simulink model "eVTOL_System"  (R2024b)
settings: Solver=FixedStepAuto  StartTime=0.0  StopTime=inf  RelTol=1e-3
undefined symbols (not defined in the file): airspeed, Battery, BCE12, BCE_Set_init, BMS_Controller_State, C, Cell10_P, Cell11_P, Cell12_P, Cell13_P, Cell14_P, Cell15_P, Cell16_P, Cell17_P, Cell18_P, Cell19_P, Cell1_N, Cell1_P, Cell20_P, Cell21_P, Cell22_P, Cell23_P, Cell24_P, Cell2_P, Cell3_P, Cell4_P, Cell5_P, Cell6_P, Cell7_P, Cell8_P, Cell9_P, Charging_State, CityMission, control, controlParams, ControlSampleTime, CriticalTiltAngle, currentFactor, CV_Gain, ddx, ddy, ddz, Device_01, Device_02, DiscIntNeverNeededParam, dx, dy, dz, Earth, env, F, F28379D_ADC_MaxCount, F28379D_ADC_Vmax, FixedWingMission, flightState, Foc_Ki_IxTcpu, Foc_Ki_S, Foc_Kp_I, Foc_Kp_S, fractalcoef ... (+68)
libraries: fl_lib x1115, nesl_utility x617, slrealtimeethercatlib x217, simulink x130, canmsglib x101, speedgoatlib_IO611_obsolete x91, slpidlib x49, mcbcontrolslib x44, slrealtimeutilitieslib x35, speedgoatlib_hdlCoder_IO3xx x31, dspstat3 x24, mcbpositiondecoderlib x12
(part 14 of 31)

== system eVTOL_System/Motor Drive/Controller1/Controller_MIL/F28379D Firmware/Phase_Current_Rescaling ==
  Ia_ADC : Inport
  Ib_ADC : Inport  Port=2
  IaOffset : Inport  Port=3
  IbOffset : Inport  Port=4
  ADCtoA : Gain  Gain=10/IO334_DAC_Vmax/IO334_iDAC_gain  RndMeth=Simplest  OutDataTypeStr=Inherit: Same as input
  Add : Sum  Inputs=+-
  Add Constant : Bias  Bias=-2^11*IO334_DAC_Vmax/F28379D_ADC_Vmax  SaturateOnIntegerOverflow=off
  Get ADC Voltage : Gain  Gain=F28379D_ADC_Vmax/F28379D_ADC_MaxCount  OutDataTypeStr=single  RndMeth=Simplest
  Mux : Mux  Inputs=2
  Mux1 : Mux  Inputs=2
  PU_Conversion : Gain  Gain=1/PU_System_I_base  RndMeth=Simplest  OutDataTypeStr=Inherit: Same as input
  Rate Transition : RateTransition
  Iab_meas_PU : Outport  VectorParamsAs1DForOutWhenUnconnected=off
  wires:
  Mux1/1 -> Rate Transition/1
  Ia_ADC/1 -> Mux/1
  Ib_ADC/1 -> Mux/2
  Mux/1 -> Add Constant/1
  PU_Conversion/1 -> Iab_meas_PU/1
  IaOffset/1 -> Mux1/1
  IbOffset/1 -> Mux1/2
  Add Constant/1 -> Get ADC Voltage/1
  Get ADC Voltage/1 -> ADCtoA/1  "Currents_inDACvoltages"
  Rate Transition/1 -> Add/2
  ADCtoA/1 -> Add/1  "Currents_A"
  Add/1 -> PU_Conversion/1  "Currents_no_offset"

== system eVTOL_System/Motor Drive/Controller1/Controller_MIL/F28379D Firmware/Speed Conditioning ==
  Spd[rpm] : Inport
  hz2pu : Gain  Gain=60/(PU_System_N_base *Maxon_645604_Np)  RndMeth=Simplest  OutDataTypeStr=Inherit: Same as input
  rads2hz : Gain  Gain=Maxon_645604_Np/(2*pi)
  rmp2rads : Gain  Gain=2*pi/60
  Spd[PU] : Outport
  wires:
  Spd[rpm]/1 -> rmp2rads/1
  rmp2rads/1 -> rads2hz/1
  rads2hz/1 -> hz2pu/1
  hz2pu/1 -> Spd[PU]/1

== system eVTOL_System/Motor Drive/Controller2/Controller_MIL/F28379D Firmware/Controller Algorithm ==
  Ia_PU : Inport
  QEP_Position_Count : Inport  Port=2
  QEP_Index_Latch : Inport  Port=3
  SpdCmd : Inport  Port=4
  Kp_S : Inport  Port=5
  Ki_S : Inport  Port=6
  EnClosedLoop : Inport  Port=7
  EnablePWM : Inport  Port=8
  Kp_i : Inport  Port=9
  Ki_ixTcpu : Inport  Port=10
  AND : Logic  IconShape=distinctive  AllPortsSameDT=off  OutDataTypeStr=boolean
  Data Type Conversion : DataTypeConversion  OutDataTypeStr=single  SaturateOnIntegerOverflow=off  RndMeth=Floor
  Demux : Demux  Outputs=2
  FOC : Subsystem
  Gain : Gain  Gain=PU_System_I_base
  Gain1 : Gain  Gain=PU_System_N_base
  Mux : Mux  Inputs=2
  Speed and Pos Decoder : Subsystem
  pmsm.PositionOffset : Constant  Value=0  SampleTime=-1
  ModWave : Outport
  PWM_Enable : Outport  Port=2
  fbk_CAN : Outport  Port=3
  wires:
  EnClosedLoop/1 -> AND/2
  Speed and Pos Decoder/1(Theta_e) -> FOC/2(Pos)
  Ia_PU/1 -> FOC/1(Iab), Gain/1
  EnablePWM/1 -> FOC/6(EnablePWM)
  Speed and Pos Decoder/3(IndexFound) -> AND/1
  AND/1 -> FOC/4(EnClosedLoop)
  pmsm.PositionOffset/1 -> Speed and Pos Decoder/3(Offset)
  Speed and Pos Decoder/2(speed) -> FOC/3(Speedfb), Gain1/1
  FOC/2(PWM_Enable) -> PWM_Enable/1
  QEP_Index_Latch/1 -> Speed and Pos Decoder/2(QEP_Index_Latch)
  FOC/1(ModWave) -> ModWave/1  "ModWave"
  Kp_S/1 -> FOC/7(Kp_S)
  Ki_S/1 -> FOC/8(Ki_S)
  SpdCmd/1 -> FOC/5(SpeedRef)
  [Speed] -> Mux/1
  [Pos] -> Mux/2
  Mux/1 -> fbk_CAN/1
  Demux/1 -> [Ia_PU]
  Demux/2 -> [Ib_PU]
  Kp_i/1 -> FOC/9(Kp_i)
  Ki_ixTcpu/1 -> FOC/10(Ki_ixTcpu)
  Gain/1 -> Demux/1
  Gain1/1 -> [Speed]
  QEP_Position_Count/1 -> Speed and Pos Decoder/1(QEP_Position_Count), Data Type Conversion/1
  Data Type Conversion/1 -> [Pos]

== system eVTOL_System/Motor Drive/Controller2/Controller_MIL/F28379D Firmware/Phase_Current_Rescaling ==
  Ia_ADC : Inport
  Ib_ADC : Inport  Port=2
  IaOffset : Inport  Port=3
  IbOffset : Inport  Port=4
  ADCtoA : Gain  Gain=10/IO334_DAC_Vmax/IO334_iDAC_gain  RndMeth=Simplest  OutDataTypeStr=Inherit: Same as input
  Add : Sum  Inputs=+-
  Add Constant : Bias  Bias=-2^11*IO334_DAC_Vmax/F28379D_ADC_Vmax  SaturateOnIntegerOverflow=off
  Get ADC Voltage : Gain  Gain=F28379D_ADC_Vmax/F28379D_ADC_MaxCount  OutDataTypeStr=single  RndMeth=Simplest
  Mux : Mux  Inputs=2
  Mux1 : Mux  Inputs=2
  PU_Conversion : Gain  Gain=1/PU_System_I_base  RndMeth=Simplest  OutDataTypeStr=Inherit: Same as input
  Rate Transition : RateTransition
  Iab_meas_PU : Outport  VectorParamsAs1DForOutWhenUnconnected=off
  wires:
  Mux1/1 -> Rate Transition/1
  Ia_ADC/1 -> Mux/1
  Ib_ADC/1 -> Mux/2
  Mux/1 -> Add Constant/1
  PU_Conversion/1 -> Iab_meas_PU/1
  IaOffset/1 -> Mux1/1
  IbOffset/1 -> Mux1/2
  Add Constant/1 -> Get ADC Voltage/1
  Get ADC Voltage/1 -> ADCtoA/1  "Currents_inDACvoltages"
  Rate Transition/1 -> Add/2
  ADCtoA/1 -> Add/1  "Currents_A"
  Add/1 -> PU_Conversion/1  "Currents_no_offset"

== system eVTOL_System/Motor Drive/Controller2/Controller_MIL/F28379D Firmware/Speed Conditioning ==
  Spd[rpm] : Inport
  hz2pu : Gain  Gain=60/(PU_System_N_base *Maxon_645604_Np)  RndMeth=Simplest  OutDataTypeStr=Inherit: Same as input
  rads2hz : Gain  Gain=Maxon_645604_Np/(2*pi)
  rmp2rads : Gain  Gain=2*pi/60
  Spd[PU] : Outport
  wires:
  Spd[rpm]/1 -> rmp2rads/1
  rmp2rads/1 -> rads2hz/1
  rads2hz/1 -> hz2pu/1
  hz2pu/1 -> Spd[PU]/1

== system eVTOL_System/Motor Drive/Controller3/Controller_MIL/F28379D Firmware/Controller Algorithm ==
  Ia_PU : Inport
  QEP_Position_Count : Inport  Port=2
  QEP_Index_Latch : Inport  Port=3
  SpdCmd : Inport  Port=4
  Kp_S : Inport  Port=5
  Ki_S : Inport  Port=6
  EnClosedLoop : Inport  Port=7
  EnablePWM : Inport  Port=8
  Kp_i : Inport  Port=9
  Ki_ixTcpu : Inport  Port=10
  AND : Logic  IconShape=distinctive  AllPortsSameDT=off  OutDataTypeStr=boolean
  Data Type Conversion : DataTypeConversion  OutDataTypeStr=single  SaturateOnIntegerOverflow=off  RndMeth=Floor
  Demux : Demux  Outputs=2
  FOC : Subsystem
  Gain : Gain  Gain=PU_System_I_base
  Gain1 : Gain  Gain=PU_System_N_base
  Mux : Mux  Inputs=2
  Speed and Pos Decoder : Subsystem
  pmsm.PositionOffset : Constant  Value=0  SampleTime=-1
  ModWave : Outport
  PWM_Enable : Outport  Port=2
  fbk_CAN : Outport  Port=3
  wires:
  EnClosedLoop/1 -> AND/2
  Speed and Pos Decoder/1(Theta_e) -> FOC/2(Pos)
  Ia_PU/1 -> FOC/1(Iab), Gain/1
  EnablePWM/1 -> FOC/6(EnablePWM)
  Speed and Pos Decoder/3(IndexFound) -> AND/1
  AND/1 -> FOC/4(EnClosedLoop)
  pmsm.PositionOffset/1 -> Speed and Pos Decoder/3(Offset)
  Speed and Pos Decoder/2(speed) -> FOC/3(Speedfb), Gain1/1
  FOC/2(PWM_Enable) -> PWM_Enable/1
  QEP_Index_Latch/1 -> Speed and Pos Decoder/2(QEP_Index_Latch)
  FOC/1(ModWave) -> ModWave/1  "ModWave"
  Kp_S/1 -> FOC/7(Kp_S)
  Ki_S/1 -> FOC/8(Ki_S)
  SpdCmd/1 -> FOC/5(SpeedRef)
  [Speed] -> Mux/1
  [Pos] -> Mux/2
  Mux/1 -> fbk_CAN/1
  Demux/1 -> [Ia_PU]
  Demux/2 -> [Ib_PU]
  Kp_i/1 -> FOC/9(Kp_i)
  Ki_ixTcpu/1 -> FOC/10(Ki_ixTcpu)
  Gain/1 -> Demux/1
  Gain1/1 -> [Speed]
  QEP_Position_Count/1 -> Speed and Pos Decoder/1(QEP_Position_Count), Data Type Conversion/1
  Data Type Conversion/1 -> [Pos]

== system eVTOL_System/Motor Drive/Controller3/Controller_MIL/F28379D Firmware/Phase_Current_Rescaling ==
  Ia_ADC : Inport
  Ib_ADC : Inport  Port=2
  IaOffset : Inport  Port=3
  IbOffset : Inport  Port=4
  ADCtoA : Gain  Gain=10/IO334_DAC_Vmax/IO334_iDAC_gain  RndMeth=Simplest  OutDataTypeStr=Inherit: Same as input
  Add : Sum  Inputs=+-
  Add Constant : Bias  Bias=-2^11*IO334_DAC_Vmax/F28379D_ADC_Vmax  SaturateOnIntegerOverflow=off
  Get ADC Voltage : Gain  Gain=F28379D_ADC_Vmax/F28379D_ADC_MaxCount  OutDataTypeStr=single  RndMeth=Simplest
  Mux : Mux  Inputs=2
  Mux1 : Mux  Inputs=2
  PU_Conversion : Gain  Gain=1/PU_System_I_base  RndMeth=Simplest  OutDataTypeStr=Inherit: Same as input
  Rate Transition : RateTransition
  Iab_meas_PU : Outport  VectorParamsAs1DForOutWhenUnconnected=off
  wires:
  Mux1/1 -> Rate Transition/1
  Ia_ADC/1 -> Mux/1
  Ib_ADC/1 -> Mux/2
  Mux/1 -> Add Constant/1
  PU_Conversion/1 -> Iab_meas_PU/1
  IaOffset/1 -> Mux1/1
  IbOffset/1 -> Mux1/2
  Add Constant/1 -> Get ADC Voltage/1
  Get ADC Voltage/1 -> ADCtoA/1  "Currents_inDACvoltages"
  Rate Transition/1 -> Add/2
  ADCtoA/1 -> Add/1  "Currents_A"
  Add/1 -> PU_Conversion/1  "Currents_no_offset"

== system eVTOL_System/Motor Drive/Controller3/Controller_MIL/F28379D Firmware/Speed Conditioning ==
  Spd[rpm] : Inport
  hz2pu : Gain  Gain=60/(PU_System_N_base *Maxon_645604_Np)  RndMeth=Simplest  OutDataTypeStr=Inherit: Same as input
  rads2hz : Gain  Gain=Maxon_645604_Np/(2*pi)
  rmp2rads : Gain  Gain=2*pi/60
  Spd[PU] : Outport
  wires:
  Spd[rpm]/1 -> rmp2rads/1
  rmp2rads/1 -> rads2hz/1
  rads2hz/1 -> hz2pu/1
  hz2pu/1 -> Spd[PU]/1

== system eVTOL_System/Motor Drive/Three-Phase PMSM Drive/PMSM and average inverter/Encoder Simulation/Get_PU  ==
  rad : Inport
  Constant2 : Constant  Value=2*pi  OutDataTypeStr=single  SampleTime=-1
  Get_PU : Gain  Gain=1/(2*pi)  RndMeth=Simplest  OutDataTypeStr=Inherit: Same as input
  Mod : Math  Operator=mod
  PU : Outport  VectorParamsAs1DForOutWhenUnconnected=off
  wires:
  Get_PU/1 -> PU/1
  Mod/1 -> Get_PU/1
  Constant2/1 -> Mod/2
  rad/1 -> Mod/1

== system eVTOL_System/Motor Drive/Three-Phase PMSM Drive/PMSM and average inverter/Encoder Simulation/Wrap ==
  in : Inport
  Constant2 : Constant  OutDataTypeStr=single  SampleTime=-1
  Mod : Math  Operator=mod
  out : Outport  VectorParamsAs1DForOutWhenUnconnected=off
  wires:
  Mod/1 -> out/1
  Constant2/1 -> Mod/2
  in/1 -> Mod/1

== system eVTOL_System/Motor Drive/Three-Phase PMSM Drive/PMSM and average inverter/Runtime to DC/To Dc A1 ==
  A_on : Inport
  A_off : Inport  Port=2
  Add : Sum
  Add Constant1 : Bias  Bias=1  SaturateOnIntegerOverflow=off
  Data Type Conversion3 : DataTypeConversion  OutDataTypeStr=double  SaturateOnIntegerOverflow=off  RndMeth=Floor
  Data Type Conversion5 : DataTypeConversion  OutDataTypeStr=double  SaturateOnIntegerOverflow=off  RndMeth=Floor
  Divide : Product  Inputs=*/
  Gain1 : Gain  Gain=-2
  Dc : Outport
  wires:
  Data Type Conversion5/1 -> Add/2
  Add Constant1/1 -> Dc/1
  Gain1/1 -> Add Constant1/1
  Add/1 -> Divide/2
  Data Type Conversion3/1 -> Add/1, Divide/1
  A_off/1 -> Data Type Conversion5/1
  Divide/1 -> Gain1/1
  A_on/1 -> Data Type Conversion3/1

== system eVTOL_System/Motor Drive/Three-Phase PMSM Drive/PMSM and average inverter/Runtime to DC/To Dc A2 ==
  A_on : Inport
  A_off : Inport  Port=2
  Add : Sum
  Add Constant1 : Bias  Bias=1  SaturateOnIntegerOverflow=off
  Data Type Conversion3 : DataTypeConversion  OutDataTypeStr=double  SaturateOnIntegerOverflow=off  RndMeth=Floor
  Data Type Conversion5 : DataTypeConversion  OutDataTypeStr=double  SaturateOnIntegerOverflow=off  RndMeth=Floor
  Divide : Product  Inputs=*/
  Gain1 : Gain  Gain=-2
  Dc : Outport
  wires:
  A_on/1 -> Data Type Conversion3/1
  Divide/1 -> Gain1/1
  A_off/1 -> Data Type Conversion5/1
  Data Type Conversion3/1 -> Divide/1, Add/1
  Add/1 -> Divide/2
  Gain1/1 -> Add Constant1/1
  Add Constant1/1 -> Dc/1
  Data Type Conversion5/1 -> Add/2

== system eVTOL_System/Motor Drive/Three-Phase PMSM Drive/PMSM and average inverter/Runtime to DC/To Dc A3 ==
  A_on : Inport
  A_off : Inport  Port=2
  Add : Sum
  Add Constant1 : Bias  Bias=1  SaturateOnIntegerOverflow=off
  Data Type Conversion3 : DataTypeConversion  OutDataTypeStr=double  SaturateOnIntegerOverflow=off  RndMeth=Floor
  Data Type Conversion5 : DataTypeConversion  OutDataTypeStr=double  SaturateOnIntegerOverflow=off  RndMeth=Floor
  Divide : Product  Inputs=*/
  Gain1 : Gain  Gain=-2
  Dc : Outport
  wires:
  Data Type Conversion5/1 -> Add/2
  Add Constant1/1 -> Dc/1
  Gain1/1 -> Add Constant1/1
  Add/1 -> Divide/2
  Data Type Conversion3/1 -> Add/1, Divide/1
  A_off/1 -> Data Type Conversion5/1
  Divide/1 -> Gain1/1
  A_on/1 -> Data Type Conversion3/1

== system eVTOL_System/Motor Drive/Three-Phase PMSM Drive/PMSM and inverter with switching dynamics/DAC Config/Subsystem ==
  Plant_frequency : Inport
  SignalFrequency : Inport  Port=2
  Add : Sum  Inputs=+-
  Data Type Conversion : DataTypeConversion  OutDataTypeStr=uint16  SaturateOnIntegerOverflow=off  RndMeth=Floor
  Divide : Product  Inputs=*/
  constant : Constant  VectorParams1D=off  SampleTime=-1
  DAC_reset : Outport
  wires:
  SignalFrequency/1 -> Divide/2
  Add/1 -> Data Type Conversion/1
  Divide/1 -> Add/1
  Data Type Conversion/1 -> DAC_reset/1
  constant/1 -> Add/2
  Plant_frequency/1 -> Divide/1

== system eVTOL_System/Motor Drive/Three-Phase PMSM Drive/PMSM and inverter with switching dynamics/Encoder Simulation/Get_PU  ==
  rad : Inport
  Constant2 : Constant  Value=2*pi  OutDataTypeStr=single  SampleTime=-1
  Get_PU : Gain  Gain=1/(2*pi)  RndMeth=Simplest  OutDataTypeStr=Inherit: Same as input
  Mod : Math  Operator=mod
  PU : Outport  VectorParamsAs1DForOutWhenUnconnected=off
  wires:
  Get_PU/1 -> PU/1
  Mod/1 -> Get_PU/1
  Constant2/1 -> Mod/2
  rad/1 -> Mod/1

== system eVTOL_System/Motor Drive/Three-Phase PMSM Drive/PMSM and inverter with switching dynamics/Encoder Simulation/Wrap ==
  in : Inport
  Constant2 : Constant  OutDataTypeStr=single  SampleTime=-1
  Mod : Math  Operator=mod
  out : Outport  VectorParamsAs1DForOutWhenUnconnected=off
  wires:
  Mod/1 -> out/1
  Constant2/1 -> Mod/2
  in/1 -> Mod/1

== system eVTOL_System/Motor Drive/Three-Phase PMSM Drive/PMSM and inverter with switching dynamics/PMSM_3P2L_Inverter_Plant_TBR/PMSM_3P2L_Inverter_Plant ==
  note: Generated by HDL Workflow Advisor on 20-Mar-2024 12:31:25
  PCIe_RC_or_TTL : Inport
  PCIe_PWM_Config : Inport  Port=2
  PCIe_PWM_Runtime : Inport  Port=3
  PCIe_PWM_Enable : Inport  Port=4
  PCIe_Protocol : Inport  Port=5
  PWM1A TTL_0 : Inport  Port=6
  PWM1B TTL_1 : Inport  Port=7
  PWM2A TTL_2 : Inport  Port=8
  PWM2B TTL_3 : Inport  Port=9
  PWM3A TTL_4 : Inport  Port=10
  PWM3B TTL_5 : Inport  Port=11
  PCIe_V_dc : Inport  Port=12
  PCIe_Fault : Inport  Port=13
  PCIe_LdTrq/Spd : Inport  Port=14
  PCIe_Motor_Config : Inport  Port=15
  PCIe_Motor_Connection : Inport  Port=16
  PCIe_QAE_Config : Inport  Port=17
  PCIe_Resolver_Config : Inport  Port=18
  PCIe_Iabc_DAC_gain : Inport  Port=19
  PCIe_Iabc_DAC_bias : Inport  Port=20
  PCIe_DAC_reset : Inport  Port=21
  AD5547 Setup : speedgoatlib_hdlCoder_IO3xx/AD5547 Setup  module_id=module_id  dacGain_1=10.0V  dacActiv_1=off  dacGain_2=2.5V  dacActiv_2=on  dacGain_3=2.5V  dacActiv_3=on  dacGain_4=2.5V  dacActiv_4=on  dacGain_5=2.5V  dacActiv_5=on  dacGain_6=10.0V  dacActiv_6=off  dacGain_7=2.5V  dacActiv_7=on  dacGain_8=10.0V  dacActiv_8=off  dacGain_9=10.0V  dacActiv_9=off  dacGain_10=10.0V  dacActiv_10=off  dacGain_11=10.0V  dacActiv_11=off  dacGain_12=10.0V  dacActiv_12=off  dacGain_13=10.0V  dacActiv_13=off  dacGain_14=10.0V  dacActiv_14=off  dacGain_15=10.0V  dacActiv_15=off  dacGain_16=10.0V  dacActiv_16=off
  DataTypeConversion{,1..4} (5 alike) : DataTypeConversion  OutDataTypeStr=fixdt(1,16,0)  ConvertRealWorld=Stored Integer (SI)  SaturateOnIntegerOverflow=off  RndMeth=Floor
  DataTypeConversion{5..10} (6 alike) : DataTypeConversion  OutDataTypeStr=fixdt('boolean')  ConvertRealWorld=Stored Integer (SI)  SaturateOnIntegerOverflow=off  RndMeth=Floor
  Ground{,1..10} (11 alike) : Ground
  IO3xx Setup : speedgoatlib_hdlCoder_IO3xx/IO3xx Setup  mdl_ss_name=PMSM3P2LInverterCHIL_limited/PMSM_3P2L_Inverter_Plant  board_type=IO334-325k  fpga_sync_mode=on  reset_mode=on  reset_mode_stop=on  device_id=1  module_id=module_id  pci_slot=slot  fpga_mat_file=c:\hdlprj\hdlsrc\PMSM3P2LInverterCHIL_limited\PMSM_3P2L_Inverter_Plant.mat  timestamp_mcs=03/20/24 12:27:31  timestamp=2403201134  tsreg=hex2dec('8')  bsf_file=PMSM_3P2L_Inverter_Plant_2403201134.mcs  mcs=0  init_reg_list=[]
  PCIRead_PCIe_Ia : speedgoatlib_hdlCoder_IO3xx/IO3xx PCI Read  device_id=1  module_id=module_id  board_type=IO334-325k  port_name=PCIe_Ia  port_offset=hex2dec('128')  port_type=single  port_dim=1  strobe=0  sample_time=ts
  PCIRead_PCIe_Ib : speedgoatlib_hdlCoder_IO3xx/IO3xx PCI Read  device_id=1  module_id=module_id  board_type=IO334-325k  port_name=PCIe_Ib  port_offset=hex2dec('12C')  port_type=single  port_dim=1  strobe=0  sample_time=ts
  PCIRead_PCIe_Ic : speedgoatlib_hdlCoder_IO3xx/IO3xx PCI Read  device_id=1  module_id=module_id  board_type=IO334-325k  port_name=PCIe_Ic  port_offset=hex2dec('130')  port_type=single  port_dim=1  strobe=0  sample_time=ts
  PCIRead_PCIe_Idc : speedgoatlib_hdlCoder_IO3xx/IO3xx PCI Read  device_id=1  module_id=module_id  board_type=IO334-325k  port_name=PCIe_Idc  port_offset=hex2dec('134')  port_type=single  port_dim=1  strobe=0  sample_time=ts
  PCIRead_PCIe_Motor_Angle : speedgoatlib_hdlCoder_IO3xx/IO3xx PCI Read  device_id=1  module_id=module_id  board_type=IO334-325k  port_name=PCIe_Motor_Angle  port_offset=hex2dec('13C')  port_type=single  port_dim=1  strobe=0  sample_time=ts
  PCIRead_PCIe_Motor_ElecAngle : speedgoatlib_hdlCoder_IO3xx/IO3xx PCI Read  device_id=1  module_id=module_id  board_type=IO334-325k  port_name=PCIe_Motor_ElecAngle  port_offset=hex2dec('184')  port_type=single  port_dim=1  strobe=0  sample_time=ts
  PCIRead_PCIe_Motor_Spd : speedgoatlib_hdlCoder_IO3xx/IO3xx PCI Read  device_id=1  module_id=module_id  board_type=IO334-325k  port_name=PCIe_Motor_Spd  port_offset=hex2dec('138')  port_type=single  port_dim=1  strobe=0  sample_time=ts
  PCIRead_PCIe_Motor_Trq : speedgoatlib_hdlCoder_IO3xx/IO3xx PCI Read  device_id=1  module_id=module_id  board_type=IO334-325k  port_name=PCIe_Motor_Trq  port_offset=hex2dec('188')  port_type=single  port_dim=1  strobe=0  sample_time=ts
  PCIRead_PCIe_Resolver_Out : speedgoatlib_hdlCoder_IO3xx/IO3xx PCI Read  device_id=1  module_id=module_id  board_type=IO334-325k  port_name=PCIe_Resolver_Out  port_offset=hex2dec('1D0')  port_type=uint32  port_dim=3  strobe=hex2dec('1E0')  sample_time=ts
  PCIRead_PCIe_Rsvl_cos_neg : speedgoatlib_hdlCoder_IO3xx/IO3xx PCI Read  device_id=1  module_id=module_id  board_type=IO334-325k  port_name=PCIe_Rsvl_cos_neg  port_offset=hex2dec('198')  port_type=uint32  port_dim=1  strobe=0  sample_time=ts
  PCIRead_PCIe_Rsvl_excitation_neg : speedgoatlib_hdlCoder_IO3xx/IO3xx PCI Read  device_id=1  module_id=module_id  board_type=IO334-325k  port_name=PCIe_Rsvl_excitation_neg  port_offset=hex2dec('190')  port_type=uint32  port_dim=1  strobe=0  sample_time=ts
  PCIRead_PCIe_Rsvl_excitation_pos : speedgoatlib_hdlCoder_IO3xx/IO3xx PCI Read  device_id=1  module_id=module_id  board_type=IO334-325k  port_name=PCIe_Rsvl_excitation_pos  port_offset=hex2dec('194')  port_type=uint32  port_dim=1  strobe=0  sample_time=ts
  PCIRead_PCIe_Rsvl_sin_neg : speedgoatlib_hdlCoder_IO3xx/IO3xx PCI Read  device_id=1  module_id=module_id  board_type=IO334-325k  port_name=PCIe_Rsvl_sin_neg  port_offset=hex2dec('18C')  port_type=uint32  port_dim=1  strobe=0  sample_time=ts
  PCIWrite_PCIe_DAC_reset : speedgoatlib_hdlCoder_IO3xx/IO3xx PCI Write  device_id=1  module_id=module_id  board_type=IO334-325k  port_name=PCIe_DAC_reset  port_offset=hex2dec('124')  port_type=uint32  port_dim=1  strobe=0  sample_time=ts
  PCIWrite_PCIe_Fault : speedgoatlib_hdlCoder_IO3xx/IO3xx PCI Write  device_id=1  module_id=module_id  board_type=IO334-325k  port_name=PCIe_Fault  port_offset=hex2dec('110')  port_type=uint32  port_dim=1  strobe=0  sample_time=ts
  PCIWrite_PCIe_Iabc_DAC_bias : speedgoatlib_hdlCoder_IO3xx/IO3xx PCI Write  device_id=1  module_id=module_id  board_type=IO334-325k  port_name=PCIe_Iabc_DAC_bias  port_offset=hex2dec('120')  port_type=single  port_dim=1  strobe=0  sample_time=ts
  PCIWrite_PCIe_Iabc_DAC_gain : speedgoatlib_hdlCoder_IO3xx/IO3xx PCI Write  device_id=1  module_id=module_id  board_type=IO334-325k  port_name=PCIe_Iabc_DAC_gain  port_offset=hex2dec('11C')  port_type=single  port_dim=1  strobe=0  sample_time=ts
  PCIWrite_PCIe_LdTrq/Spd : speedgoatlib_hdlCoder_IO3xx/IO3xx PCI Write  device_id=1  module_id=module_id  board_type=IO334-325k  port_name=PCIe_LdTrq//Spd  port_offset=hex2dec('114')  port_type=single  port_dim=1  strobe=0  sample_time=ts
  PCIWrite_PCIe_Motor_Config : speedgoatlib_hdlCoder_IO3xx/IO3xx PCI Write  device_id=1  module_id=module_id  board_type=IO334-325k  port_name=PCIe_Motor_Config  port_offset=hex2dec('340')  port_type=single  port_dim=9  strobe=hex2dec('380')  sample_time=ts
  PCIWrite_PCIe_Motor_Connection : speedgoatlib_hdlCoder_IO3xx/IO3xx PCI Write  device_id=1  module_id=module_id  board_type=IO334-325k  port_name=PCIe_Motor_Connection  port_offset=hex2dec('118')  port_type=uint32  port_dim=1  strobe=0  sample_time=ts
  PCIWrite_PCIe_PWM_Config : speedgoatlib_hdlCoder_IO3xx/IO3xx PCI Write  device_id=1  module_id=module_id  board_type=IO334-325k  port_name=PCIe_PWM_Config  port_offset=hex2dec('200')  port_type=uint32  port_dim=48  strobe=hex2dec('300')  sample_time=ts
  PCIWrite_PCIe_PWM_Enable : speedgoatlib_hdlCoder_IO3xx/IO3xx PCI Write  device_id=1  module_id=module_id  board_type=IO334-325k  port_name=PCIe_PWM_Enable  port_offset=hex2dec('104')  port_type=uint32  port_dim=1  strobe=0  sample_time=ts
  PCIWrite_PCIe_PWM_Runtime : speedgoatlib_hdlCoder_IO3xx/IO3xx PCI Write  device_id=1  module_id=module_id  board_type=IO334-325k  port_name=PCIe_PWM_Runtime  port_offset=hex2dec('140')  port_type=uint32  port_dim=15  strobe=hex2dec('180')  sample_time=ts
  PCIWrite_PCIe_Protocol : speedgoatlib_hdlCoder_IO3xx/IO3xx PCI Write  device_id=1  module_id=module_id  board_type=IO334-325k  port_name=PCIe_Protocol  port_offset=hex2dec('108')  port_type=uint32  port_dim=1  strobe=0  sample_time=ts
  PCIWrite_PCIe_QAE_Config : speedgoatlib_hdlCoder_IO3xx/IO3xx PCI Write  device_id=1  module_id=module_id  board_type=IO334-325k  port_name=PCIe_QAE_Config  port_offset=hex2dec('3C0')  port_type=uint32  port_dim=8  strobe=hex2dec('3E0')  sample_time=ts
  PCIWrite_PCIe_RC_or_TTL : speedgoatlib_hdlCoder_IO3xx/IO3xx PCI Write  device_id=1  module_id=module_id  board_type=IO334-325k  port_name=PCIe_RC_or_TTL  port_offset=hex2dec('100')  port_type=uint32  port_dim=1  strobe=0  sample_time=ts
  PCIWrite_PCIe_Resolver_Config : speedgoatlib_hdlCoder_IO3xx/IO3xx PCI Write  device_id=1  module_id=module_id  board_type=IO334-325k  port_name=PCIe_Resolver_Config  port_offset=hex2dec('480')  port_type=uint32  port_dim=17  strobe=hex2dec('500')  sample_time=ts
  PCIWrite_PCIe_V_dc : speedgoatlib_hdlCoder_IO3xx/IO3xx PCI Write  device_id=1  module_id=module_id  board_type=IO334-325k  port_name=PCIe_V_dc  port_offset=hex2dec('10C')  port_type=single  port_dim=1  strobe=0  sample_time=ts
  Port Settings -2x 0x00590000 : speedgoatlib_hdlCoder_IO3xx/Port Settings -2x  module_id=module_id  rearIO=-21  PullRPort0=pull-up 3.3V  VioPort0=3.3V  PullRPort1=pull-up 3.3V  VioPort1=3.3V  PullRPort2=pull-up 3.3V  VioPort2=3.3V  PullRPort3=pull-up 3.3V  VioPort3=3.3V  PullRPort4=pull-up 3.3V  VioPort4=3.3V  PullRPort5=pull-up 3.3V  VioPort5=3.3V  PullRPort6=pull-up 3.3V  VioPort6=3.3V  I2cAddrOffset=5832704  DutAddrOffset=120
  Terminator{,1..5} (6 alike) : Terminator
  dtc{,1..9} (10 alike) : DataTypeConversion  OutDataTypeStr=uint32  ConvertRealWorld=Stored Integer (SI)  SaturateOnIntegerOverflow=off
  dtc{10..13} (4 alike) : DataTypeConversion  OutDataTypeStr=fixdt(1,16,0)  ConvertRealWorld=Stored Integer (SI)  SaturateOnIntegerOverflow=off
  dtc14 : DataTypeConversion  OutDataTypeStr=fixdt(0,32,0)  ConvertRealWorld=Stored Integer (SI)  SaturateOnIntegerOverflow=off
  sSpec{,3..4,6} (4 alike) : SignalSpecification  OutDataTypeStr=fixdt('boolean')
  sSpec{1,5,7..8} (4 alike) : SignalSpecification  OutDataTypeStr=fixdt(0,32,0)
  sSpec2 : SignalSpecification  OutDataTypeStr=fixdt(0,24,0)
  sSpec9 : SignalSpecification  OutDataTypeStr=fixdt(0,16,0)
  PCIe_Ia : Outport
  PCIe_Ib : Outport  Port=2
  PCIe_Ic : Outport  Port=3
  AO_2_Ia : Outport  Port=4
  AO_3_Ib : Outport  Port=5
  AO_4_Ic : Outport  Port=6
  PCIe_Idc : Outport  Port=7
  PCIe_Motor_Spd : Outport  Port=8
  PCIe_Motor_Angle : Outport  Port=9
  PCIe_Motor_ElecAngle : Outport  Port=10
  PCIe_Motor_Trq : Outport  Port=11
  TTL_48_QEP_A_A : Outport  Port=12
  TTL_49_QEP_A_B : Outport  Port=13
  "TTL_50_QEP_A_I   " : Outport  Port=14
  PCIe_Rsvl_excitation_pos : Outport  Port=15
  PCIe_Rsvl_excitation_neg : Outport  Port=16
  AO_5_Rsvl_sin_pos : Outport  Port=17
  PCIe_Rsvl_sin_neg : Outport  Port=18
  AO_7_Rsvl_cos_pos : Outport  Port=19
  PCIe_Rsvl_cos_neg : Outport  Port=20
  PCIe_Resolver_Out : Outport  Port=21
  TTL_32_Protocol : Outport  Port=22
  TTL_24_AO_trigger_1_8 : Outport  Port=23
  1_8_Null_AO_trigger : Outport  Port=24
  wires:
  PCIe_RC_or_TTL/1 -> sSpec/1
  sSpec/1 -> dtc/1
  dtc/1 -> PCIWrite_PCIe_RC_or_TTL/1
  PCIe_PWM_Config/1 -> sSpec1/1
  sSpec1/1 -> dtc1/1
  dtc1/1 -> PCIWrite_PCIe_PWM_Config/1
  PCIe_PWM_Runtime/1 -> sSpec2/1
  sSpec2/1 -> dtc2/1
  dtc2/1 -> PCIWrite_PCIe_PWM_Runtime/1
  PCIe_PWM_Enable/1 -> sSpec3/1
  sSpec3/1 -> dtc3/1
  dtc3/1 -> PCIWrite_PCIe_PWM_Enable/1
  PCIe_Protocol/1 -> sSpec4/1
  sSpec4/1 -> dtc4/1
  dtc4/1 -> PCIWrite_PCIe_Protocol/1
  PCIe_V_dc/1 -> PCIWrite_PCIe_V_dc/1
  PCIe_Fault/1 -> sSpec5/1
  sSpec5/1 -> dtc5/1
  dtc5/1 -> PCIWrite_PCIe_Fault/1
  PCIe_LdTrq/Spd/1 -> PCIWrite_PCIe_LdTrq/Spd/1
  PCIe_Motor_Config/1 -> PCIWrite_PCIe_Motor_Config/1
  PCIe_Motor_Connection/1 -> sSpec6/1
  sSpec6/1 -> dtc6/1
  dtc6/1 -> PCIWrite_PCIe_Motor_Connection/1
  PCIe_QAE_Config/1 -> sSpec7/1
  sSpec7/1 -> dtc7/1
  dtc7/1 -> PCIWrite_PCIe_QAE_Config/1
  PCIe_Resolver_Config/1 -> sSpec8/1
  sSpec8/1 -> dtc8/1
  dtc8/1 -> PCIWrite_PCIe_Resolver_Config/1
  PCIe_Iabc_DAC_gain/1 -> PCIWrite_PCIe_Iabc_DAC_gain/1
  PCIe_Iabc_DAC_bias/1 -> PCIWrite_PCIe_Iabc_DAC_bias/1
  PCIe_DAC_reset/1 -> sSpec9/1
  sSpec9/1 -> dtc9/1
  dtc9/1 -> PCIWrite_PCIe_DAC_reset/1
  PCIRead_PCIe_Ia/1 -> PCIe_Ia/1
  PCIRead_PCIe_Ib/1 -> PCIe_Ib/1
  PCIRead_PCIe_Ic/1 -> PCIe_Ic/1
  PCIRead_PCIe_Idc/1 -> PCIe_Idc/1
  PCIRead_PCIe_Motor_Spd/1 -> PCIe_Motor_Spd/1
  PCIRead_PCIe_Motor_Angle/1 -> PCIe_Motor_Angle/1
  PCIRead_PCIe_Motor_ElecAngle/1 -> PCIe_Motor_ElecAngle/1
  PCIRead_PCIe_Motor_Trq/1 -> PCIe_Motor_Trq/1
  dtc10/1 -> PCIe_Rsvl_excitation_pos/1
  PCIRead_PCIe_Rsvl_excitation_pos/1 -> dtc10/1
  dtc11/1 -> PCIe_Rsvl_excitation_neg/1
  PCIRead_PCIe_Rsvl_excitation_neg/1 -> dtc11/1
  dtc12/1 -> PCIe_Rsvl_sin_neg/1
  PCIRead_PCIe_Rsvl_sin_neg/1 -> dtc12/1
  dtc13/1 -> PCIe_Rsvl_cos_neg/1
  PCIRead_PCIe_Rsvl_cos_neg/1 -> dtc13/1
  dtc14/1 -> PCIe_Resolver_Out/1
  PCIRead_PCIe_Resolver_Out/1 -> dtc14/1
  DataTypeConversion/1 -> AO_2_Ia/1
  Ground/1 -> DataTypeConversion/1
  DataTypeConversion1/1 -> AO_3_Ib/1
  Ground1/1 -> DataTypeConversion1/1
  DataTypeConversion2/1 -> AO_4_Ic/1
  Ground2/1 -> DataTypeConversion2/1
  DataTypeConversion3/1 -> AO_5_Rsvl_sin_pos/1
  Ground3/1 -> DataTypeConversion3/1
  DataTypeConversion4/1 -> AO_7_Rsvl_cos_pos/1
  Ground4/1 -> DataTypeConversion4/1
  DataTypeConversion5/1 -> 1_8_Null_AO_trigger/1
  Ground5/1 -> DataTypeConversion5/1
  PWM1A TTL_0/1 -> Terminator/1
  PWM1B TTL_1/1 -> Terminator1/1
  PWM2A TTL_2/1 -> Terminator2/1
  PWM2B TTL_3/1 -> Terminator3/1
  PWM3A TTL_4/1 -> Terminator4/1
  PWM3B TTL_5/1 -> Terminator5/1
  DataTypeConversion6/1 -> TTL_48_QEP_A_A/1
  Ground6/1 -> DataTypeConversion6/1
  DataTypeConversion7/1 -> TTL_49_QEP_A_B/1
  Ground7/1 -> DataTypeConversion7/1
  DataTypeConversion8/1 -> "TTL_50_QEP_A_I   "/1
  Ground8/1 -> DataTypeConversion8/1
  DataTypeConversion9/1 -> TTL_32_Protocol/1
  Ground9/1 -> DataTypeConversion9/1
  DataTypeConversion10/1 -> TTL_24_AO_trigger_1_8/1
  Ground10/1 -> DataTypeConversion10/1

== system eVTOL_System/Motor Drive/Three-Phase PMSM Drive1/PMSM and average inverter/Encoder Simulation/Get_PU  ==
  rad : Inport
  Constant2 : Constant  Value=2*pi  OutDataTypeStr=single  SampleTime=-1
  Get_PU : Gain  Gain=1/(2*pi)  RndMeth=Simplest  OutDataTypeStr=Inherit: Same as input
  Mod : Math  Operator=mod
  PU : Outport  VectorParamsAs1DForOutWhenUnconnected=off
  wires:
  Get_PU/1 -> PU/1
  Mod/1 -> Get_PU/1
  Constant2/1 -> Mod/2
  rad/1 -> Mod/1

== system eVTOL_System/Motor Drive/Three-Phase PMSM Drive1/PMSM and average inverter/Encoder Simulation/Wrap ==
  in : Inport
  Constant2 : Constant  OutDataTypeStr=single  SampleTime=-1
  Mod : Math  Operator=mod
  out : Outport  VectorParamsAs1DForOutWhenUnconnected=off
  wires:
  Mod/1 -> out/1
  Constant2/1 -> Mod/2
  in/1 -> Mod/1

== system eVTOL_System/Motor Drive/Three-Phase PMSM Drive1/PMSM and average inverter/Runtime to DC/To Dc A1 ==
  A_on : Inport
  A_off : Inport  Port=2
  Add : Sum
  Add Constant1 : Bias  Bias=1  SaturateOnIntegerOverflow=off
  Data Type Conversion3 : DataTypeConversion  OutDataTypeStr=double  SaturateOnIntegerOverflow=off  RndMeth=Floor
  Data Type Conversion5 : DataTypeConversion  OutDataTypeStr=double  SaturateOnIntegerOverflow=off  RndMeth=Floor
  Divide : Product  Inputs=*/
  Gain1 : Gain  Gain=-2
  Dc : Outport
  wires:
  Data Type Conversion5/1 -> Add/2
  Add Constant1/1 -> Dc/1
  Gain1/1 -> Add Constant1/1
  Add/1 -> Divide/2
  Data Type Conversion3/1 -> Add/1, Divide/1
  A_off/1 -> Data Type Conversion5/1
  Divide/1 -> Gain1/1
  A_on/1 -> Data Type Conversion3/1

== system eVTOL_System/Motor Drive/Three-Phase PMSM Drive1/PMSM and average inverter/Runtime to DC/To Dc A2 ==
  A_on : Inport
  A_off : Inport  Port=2
  Add : Sum
  Add Constant1 : Bias  Bias=1  SaturateOnIntegerOverflow=off
  Data Type Conversion3 : DataTypeConversion  OutDataTypeStr=double  SaturateOnIntegerOverflow=off  RndMeth=Floor
  Data Type Conversion5 : DataTypeConversion  OutDataTypeStr=double  SaturateOnIntegerOverflow=off  RndMeth=Floor
  Divide : Product  Inputs=*/
  Gain1 : Gain  Gain=-2
  Dc : Outport
  wires:
  A_on/1 -> Data Type Conversion3/1
  Divide/1 -> Gain1/1
  A_off/1 -> Data Type Conversion5/1
  Data Type Conversion3/1 -> Divide/1, Add/1
  Add/1 -> Divide/2
  Gain1/1 -> Add Constant1/1
  Add Constant1/1 -> Dc/1
  Data Type Conversion5/1 -> Add/2

== system eVTOL_System/Motor Drive/Three-Phase PMSM Drive1/PMSM and average inverter/Runtime to DC/To Dc A3 ==
  A_on : Inport
  A_off : Inport  Port=2
  Add : Sum
  Add Constant1 : Bias  Bias=1  SaturateOnIntegerOverflow=off
  Data Type Conversion3 : DataTypeConversion  OutDataTypeStr=double  SaturateOnIntegerOverflow=off  RndMeth=Floor
  Data Type Conversion5 : DataTypeConversion  OutDataTypeStr=double  SaturateOnIntegerOverflow=off  RndMeth=Floor
  Divide : Product  Inputs=*/
  Gain1 : Gain  Gain=-2
  Dc : Outport
  wires:
  Data Type Conversion5/1 -> Add/2
  Add Constant1/1 -> Dc/1
  Gain1/1 -> Add Constant1/1
  Add/1 -> Divide/2
  Data Type Conversion3/1 -> Add/1, Divide/1
  A_off/1 -> Data Type Conversion5/1
  Divide/1 -> Gain1/1
  A_on/1 -> Data Type Conversion3/1

== system eVTOL_System/Motor Drive/Three-Phase PMSM Drive2/PMSM and average inverter/Encoder Simulation/Get_PU  ==
  rad : Inport
  Constant2 : Constant  Value=2*pi  OutDataTypeStr=single  SampleTime=-1
  Get_PU : Gain  Gain=1/(2*pi)  RndMeth=Simplest  OutDataTypeStr=Inherit: Same as input
  Mod : Math  Operator=mod
  PU : Outport  VectorParamsAs1DForOutWhenUnconnected=off
  wires:
  Get_PU/1 -> PU/1
  Mod/1 -> Get_PU/1
  Constant2/1 -> Mod/2
  rad/1 -> Mod/1

== system eVTOL_System/Motor Drive/Three-Phase PMSM Drive2/PMSM and average inverter/Encoder Simulation/Wrap ==
  in : Inport
  Constant2 : Constant  OutDataTypeStr=single  SampleTime=-1
  Mod : Math  Operator=mod
  out : Outport  VectorParamsAs1DForOutWhenUnconnected=off
  wires:
  Mod/1 -> out/1
  Constant2/1 -> Mod/2
  in/1 -> Mod/1

== system eVTOL_System/Motor Drive/Three-Phase PMSM Drive2/PMSM and average inverter/Runtime to DC/To Dc A1 ==
  A_on : Inport
  A_off : Inport  Port=2
  Add : Sum
  Add Constant1 : Bias  Bias=1  SaturateOnIntegerOverflow=off
  Data Type Conversion3 : DataTypeConversion  OutDataTypeStr=double  SaturateOnIntegerOverflow=off  RndMeth=Floor
  Data Type Conversion5 : DataTypeConversion  OutDataTypeStr=double  SaturateOnIntegerOverflow=off  RndMeth=Floor
  Divide : Product  Inputs=*/
  Gain1 : Gain  Gain=-2
  Dc : Outport
  wires:
  Data Type Conversion5/1 -> Add/2
  Add Constant1/1 -> Dc/1
  Gain1/1 -> Add Constant1/1
  Add/1 -> Divide/2
  Data Type Conversion3/1 -> Add/1, Divide/1
  A_off/1 -> Data Type Conversion5/1
  Divide/1 -> Gain1/1
  A_on/1 -> Data Type Conversion3/1

== system eVTOL_System/Motor Drive/Three-Phase PMSM Drive2/PMSM and average inverter/Runtime to DC/To Dc A2 ==
  A_on : Inport
  A_off : Inport  Port=2
  Add : Sum
  Add Constant1 : Bias  Bias=1  SaturateOnIntegerOverflow=off
  Data Type Conversion3 : DataTypeConversion  OutDataTypeStr=double  SaturateOnIntegerOverflow=off  RndMeth=Floor
  Data Type Conversion5 : DataTypeConversion  OutDataTypeStr=double  SaturateOnIntegerOverflow=off  RndMeth=Floor
  Divide : Product  Inputs=*/
  Gain1 : Gain  Gain=-2
  Dc : Outport
  wires:
  A_on/1 -> Data Type Conversion3/1
  Divide/1 -> Gain1/1
  A_off/1 -> Data Type Conversion5/1
  Data Type Conversion3/1 -> Divide/1, Add/1
  Add/1 -> Divide/2
  Gain1/1 -> Add Constant1/1
  Add Constant1/1 -> Dc/1
  Data Type Conversion5/1 -> Add/2

== system eVTOL_System/Motor Drive/Three-Phase PMSM Drive2/PMSM and average inverter/Runtime to DC/To Dc A3 ==
  A_on : Inport
  A_off : Inport  Port=2
  Add : Sum
  Add Constant1 : Bias  Bias=1  SaturateOnIntegerOverflow=off
  Data Type Conversion3 : DataTypeConversion  OutDataTypeStr=double  SaturateOnIntegerOverflow=off  RndMeth=Floor
  Data Type Conversion5 : DataTypeConversion  OutDataTypeStr=double  SaturateOnIntegerOverflow=off  RndMeth=Floor
  Divide : Product  Inputs=*/
  Gain1 : Gain  Gain=-2
  Dc : Outport
  wires:
  Data Type Conversion5/1 -> Add/2
  Add Constant1/1 -> Dc/1
  Gain1/1 -> Add Constant1/1
  Add/1 -> Divide/2
  Data Type Conversion3/1 -> Add/1, Divide/1
  A_off/1 -> Data Type Conversion5/1
  Divide/1 -> Gain1/1
  A_on/1 -> Data Type Conversion3/1

== system eVTOL_System/Motor Drive/Three-Phase PMSM Drive3/PMSM and average inverter/Encoder Simulation/Get_PU  ==
  rad : Inport
  Constant2 : Constant  Value=2*pi  OutDataTypeStr=single  SampleTime=-1
  Get_PU : Gain  Gain=1/(2*pi)  RndMeth=Simplest  OutDataTypeStr=Inherit: Same as input
  Mod : Math  Operator=mod
  PU : Outport  VectorParamsAs1DForOutWhenUnconnected=off
  wires:
  Get_PU/1 -> PU/1
  Mod/1 -> Get_PU/1
  Constant2/1 -> Mod/2
  rad/1 -> Mod/1

== system eVTOL_System/Motor Drive/Three-Phase PMSM Drive3/PMSM and average inverter/Encoder Simulation/Wrap ==
  in : Inport
  Constant2 : Constant  OutDataTypeStr=single  SampleTime=-1
  Mod : Math  Operator=mod
  out : Outport  VectorParamsAs1DForOutWhenUnconnected=off
  wires:
  Mod/1 -> out/1
  Constant2/1 -> Mod/2
  in/1 -> Mod/1

== system eVTOL_System/Motor Drive/Three-Phase PMSM Drive3/PMSM and average inverter/Runtime to DC/To Dc A1 ==
  A_on : Inport
  A_off : Inport  Port=2
  Add : Sum
  Add Constant1 : Bias  Bias=1  SaturateOnIntegerOverflow=off
  Data Type Conversion3 : DataTypeConversion  OutDataTypeStr=double  SaturateOnIntegerOverflow=off  RndMeth=Floor
  Data Type Conversion5 : DataTypeConversion  OutDataTypeStr=double  SaturateOnIntegerOverflow=off  RndMeth=Floor
  Divide : Product  Inputs=*/
  Gain1 : Gain  Gain=-2
  Dc : Outport
  wires:
  Data Type Conversion5/1 -> Add/2
  Add Constant1/1 -> Dc/1
  Gain1/1 -> Add Constant1/1
  Add/1 -> Divide/2
  Data Type Conversion3/1 -> Add/1, Divide/1
  A_off/1 -> Data Type Conversion5/1
  Divide/1 -> Gain1/1
  A_on/1 -> Data Type Conversion3/1

== system eVTOL_System/Motor Drive/Three-Phase PMSM Drive3/PMSM and average inverter/Runtime to DC/To Dc A2 ==
  A_on : Inport
  A_off : Inport  Port=2
  Add : Sum
  Add Constant1 : Bias  Bias=1  SaturateOnIntegerOverflow=off
  Data Type Conversion3 : DataTypeConversion  OutDataTypeStr=double  SaturateOnIntegerOverflow=off  RndMeth=Floor
  Data Type Conversion5 : DataTypeConversion  OutDataTypeStr=double  SaturateOnIntegerOverflow=off  RndMeth=Floor
  Divide : Product  Inputs=*/
  Gain1 : Gain  Gain=-2
  Dc : Outport
  wires:
  A_on/1 -> Data Type Conversion3/1
  Divide/1 -> Gain1/1
  A_off/1 -> Data Type Conversion5/1
  Data Type Conversion3/1 -> Divide/1, Add/1
  Add/1 -> Divide/2
  Gain1/1 -> Add Constant1/1
  Add Constant1/1 -> Dc/1
  Data Type Conversion5/1 -> Add/2

== system eVTOL_System/Motor Drive/Three-Phase PMSM Drive3/PMSM and average inverter/Runtime to DC/To Dc A3 ==
  A_on : Inport
  A_off : Inport  Port=2
  Add : Sum
  Add Constant1 : Bias  Bias=1  SaturateOnIntegerOverflow=off
  Data Type Conversion3 : DataTypeConversion  OutDataTypeStr=double  SaturateOnIntegerOverflow=off  RndMeth=Floor
  Data Type Conversion5 : DataTypeConversion  OutDataTypeStr=double  SaturateOnIntegerOverflow=off  RndMeth=Floor
  Divide : Product  Inputs=*/
  Gain1 : Gain  Gain=-2
  Dc : Outport
  wires:
  Data Type Conversion5/1 -> Add/2
  Add Constant1/1 -> Dc/1
  Gain1/1 -> Add Constant1/1
  Add/1 -> Divide/2
  Data Type Conversion3/1 -> Add/1, Divide/1
  A_off/1 -> Data Type Conversion5/1
  Divide/1 -> Gain1/1
  A_on/1 -> Data Type Conversion3/1
